simulink model "RefModel_compass"  (R2020b)
settings: Solver=FixedStepDiscrete  StartTime=0.0  StopTime=inf  FixedStep=Ts_Compass.Ts_base  RelTol=1e-3
libraries: aerolibobsolete x1
settings Model: Creator=sl  LastModifiedBy=sl
settings OptimizationCC: DefaultParameterBehavior=Inlined  EnhancedBackFolding=on  PassReuseOutputArgsAs=Individual arguments  ZeroExternalMemoryAtStartup=off  ZeroInternalMemoryAtStartup=off  OptimizeBlockOrder=speed  DifferentSizesBufferReuse=on  OptimizationCustomize=off  EfficientTunableParamExpr=on
settings DebuggingCC: ParameterTunabilityLossMsg=error
settings SFSimCC: MATLABDynamicMemAlloc=off
settings RTWCC: Description=Embedded Coder  SystemTargetFile=ert.tlc  TemplateMakefile=ert_default_tmf  GenerateReport=on  IncludeHyperlinkInReport=on  LaunchReport=on  GenerateTraceInfo=on  GenerateTraceReport=on  GenerateTraceReportSl=on  GenerateTraceReportSf=on  GenerateTraceReportEml=on
settings CodeAppCC: ForceParamTrailComments=on  IgnoreCustomStorageClasses=off  OperatorAnnotations=on  SimulinkDataObjDesc=on  SFDataObjDesc=on  InsertBlockDesc=on
settings ERTTargetCC: TargetLangStandard=C99 (ISO)  GenerateSampleERTMain=on  InlinedParameterPlacement=NonHierarchical  ERTCustomFileTemplate=example_file_process.tlc

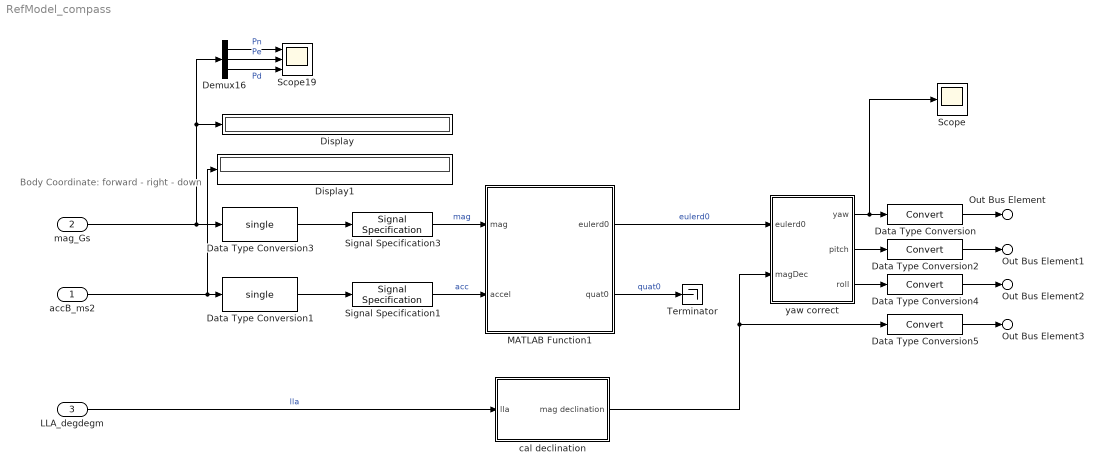
== system RefModel_compass ==
  note: Body Coordinate: forward - right - down
  accB_ms2 : Inport  PortDimensions=[1,3]
  mag_Gs : Inport  Port=2  PortDimensions=[1,3]
  LLA_degdegm : Inport  Port=3  PortDimensions=[1,3]
  Data Type Conversion{,2,4..5} (4 alike) : DataTypeConversion
  Data Type Conversion1 : DataTypeConversion  OutDataTypeStr=single
  Data Type Conversion3 : DataTypeConversion  OutDataTypeStr=single
  Demux16 : Demux  Outputs=3
  Display : Display
  Display1 : Display
  MATLAB Function1 : MATLAB Function  TreatAsAtomicUnit=on
  Scope : Scope
  Scope19 : Scope  NumInputPorts=3
  Signal Specification1 : SignalSpecification  Dimensions=[1,3]
  Signal Specification3 : SignalSpecification  Dimensions=[1,3]
  Terminator : Terminator
  cal declination : Subsystem
  yaw correct : Subsystem
  Out Bus Element : Outport  PortName=ecompass_out  Element=compass_yawd
  Out Bus Element1 : Outport  PortName=ecompass_out  Element=compass_pitchd
  Out Bus Element2 : Outport  PortName=ecompass_out  Element=compass_rolld
  Out Bus Element3 : Outport  PortName=ecompass_out  Element=compass_magDeclinationd
  wires:
  MATLAB Function1/1(eulerd0) -> yaw correct/1(eulerd0)  "eulerd0"
  Demux16/3 -> Scope19/3  "Pd"
  accB_ms2/1 -> Display1/1, Data Type Conversion1/1
  yaw correct/1(yaw) -> Data Type Conversion/1, Scope/1
  Signal Specification3/1 -> MATLAB Function1/1(mag)  "mag"
  LLA_degdegm/1 -> cal declination/1(lla)  "lla"
  Demux16/1 -> Scope19/1  "Pn"
  Signal Specification1/1 -> MATLAB Function1/2(accel)  "acc"
  Data Type Conversion3/1 -> Signal Specification3/1
  yaw correct/3(roll) -> Data Type Conversion4/1
  MATLAB Function1/2(quat0) -> Terminator/1  "quat0"
  yaw correct/2(pitch) -> Data Type Conversion2/1
  Data Type Conversion/1 -> Out Bus Element/1
  Demux16/2 -> Scope19/2  "Pe"
  Data Type Conversion1/1 -> Signal Specification1/1
  mag_Gs/1 -> Demux16/1, Display/1, Data Type Conversion3/1
  cal declination/1(mag declination) -> Data Type Conversion5/1, yaw correct/2(magDec)
  Data Type Conversion2/1 -> Out Bus Element1/1
  Data Type Conversion4/1 -> Out Bus Element2/1
  Data Type Conversion5/1 -> Out Bus Element3/1

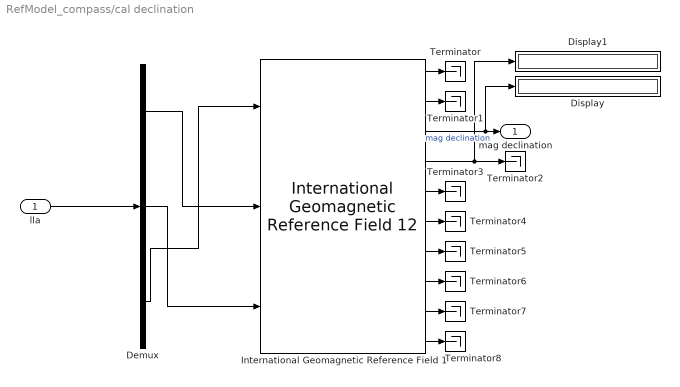
== system RefModel_compass/cal declination ==
  lla : Inport
  Demux : Demux  Outputs=3
  Display : Display
  Display1 : Display
  International Geomagnetic Reference Field 1 : aerolibobsolete/International Geomagnetic Reference Field 12  units=Metric (MKS)  time_in=off  month=January  day=1  year=2020  action=None  sv_out=on
      settings: SourceProductBaseCode=AE
  Terminator{,1..8} (9 alike) : Terminator
  mag declination : Outport
  wires:
  Demux/3 -> International Geomagnetic Reference Field 1/1
  Demux/1 -> International Geomagnetic Reference Field 1/2
  International Geomagnetic Reference Field 1/9 -> Terminator7/1
  International Geomagnetic Reference Field 1/10 -> Terminator8/1
  International Geomagnetic Reference Field 1/4 -> Display1/1, Terminator2/1
  International Geomagnetic Reference Field 1/1 -> Terminator/1
  Demux/2 -> International Geomagnetic Reference Field 1/3
  International Geomagnetic Reference Field 1/2 -> Terminator1/1
  International Geomagnetic Reference Field 1/3 -> Display/1, mag declination/1  "mag declination"
  International Geomagnetic Reference Field 1/5 -> Terminator3/1
  International Geomagnetic Reference Field 1/6 -> Terminator4/1
  International Geomagnetic Reference Field 1/8 -> Terminator6/1
  International Geomagnetic Reference Field 1/7 -> Terminator5/1
  lla/1 -> Demux/1

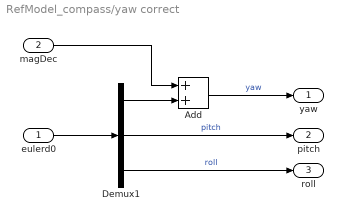
== system RefModel_compass/yaw correct ==
  eulerd0 : Inport
  magDec : Inport  Port=2
  Add : Sum
  Demux1 : Demux  Outputs=3
  yaw : Outport
  pitch : Outport  Port=2
  roll : Outport  Port=3
  wires:
  magDec/1 -> Add/1
  eulerd0/1 -> Demux1/1
  Demux1/2 -> pitch/1  "pitch"
  Demux1/3 -> roll/1  "roll"
  Demux1/1 -> Add/2
  Add/1 -> yaw/1  "yaw"

== matlab function RefModel_compass/MATLAB Function1 ==
  data: mag input; accel input; eulerd0 output; quat0 output
function [eulerd0,quat0] = compass(mag,accel)
    quat0 = single(zeros(1,4));
    eulerd0 = single(zeros(1,3));
    quat0 = compact(ecompass(accel,mag));
    eulerd0 = eulerd(quat0);
end


function eout = eulerd(quat)
% rotate 'ZYX'
qa = quat(1);
qb = quat(2);
qc = quat(3);
qd = quat(4);
the1 = single(1);
the2 = single(2);

tmp = qb.*qd.*the2 - qa.*qc.*the2;
if tmp > the1
    tmp = the1;
elseif tmp < -the1
    tmp = -the1;
end
% tmp(tmp > the1) = the1;
% tmp(tmp < -the1) = -the1;
b = -asin(tmp);
a = atan2((qa.*qd.*the2 + qb.*qc.*the2),(qa.^2.*the2 - the1 + qb.^2.*the2));
c = atan2((qa.*qb.*the2 + qc.*qd.*the2),(qa.^2.*the2 - the1 + qd.^2.*the2));
eout = [a b c]*180/pi;
end

% 
% function [eulerd0,quat0] = compass(i,accel,mag,imuUpdateFs,magUpdateFs)
%     fs = imuUpdateFs;
%     quat0 = zeros(1,4);
%     eulerd0 = zeros(1,3);
%     if rem(i,fs/magUpdateFs) == 0 && i ~= 1
%         quat0 = compact(ecompass(accel,mag));
%         eulerd0 = eulerd(quat0);
%     end
% end
